simulink model "c00008_harness"  (R2018a)
settings: Solver=FixedStepAuto  StartTime=0  StopTime=300  FixedStep=0.01  RelTol=1e-3
undefined symbols (not defined in the file): sigbuilder_block
settings Model: SldvGeneratedHarnessModel=TestUnitModel=Tanks150|  Creator=aarrieta  LastModifiedBy=umarkiegi
settings DataIOCC: ExternalInput=externalinputdata  SaveFormat=StructureWithTime
settings DebuggingCC: InheritedTsInSrcMsg=none
settings ConfigComp: CovEnable=on  CovScope=ReferencedModels  RecordCoverage=on  CovMetricSettings=dcmobe  CovHTMLOptions=-aTS=1 -bRG=1 -bTC=0 -hTR=0 -nFC=0 -scm=1 -bcm=1  CovHtmlReporting=on

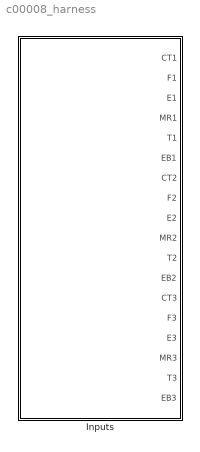
== system c00008_harness ==
  Inputs : Subsystem  Tag=STV Subsys  LoadFcn=sigbuilder_block('load');  StartFcn=sigbuilder_block('start');  StopFcn=sigbuilder_block('stop');  ClipboardFcn=sigbuilder_block('clipboard');  mask(Sigbuilder block){tuvar=[0:10]}
      mask init:
      | if ~strcmp(get_param(bdroot(gcb),'SimulationStatus'),'stopped'),tuvar = sigbuilder_block('maskInit'); end
      settings: CopyFcn=sigbuilder_block('copy');  DeleteFcn=sigbuilder_block('delete');  ModelCloseFcn=sigbuilder_block('modelClose');  PreSaveFcn=sigbuilder_block('preSave');  PauseFcn=sigbuilder_block('pause');  ContinueFcn=sigbuilder_block('continue');  NameChangeFcn=sigbuilder_block('namechange');  OpenFcn=sigbuilder_block('open',[276.75 163.5 675.75 486.75 ]);  CloseFcn=sigbuilder_block('close');
      mask Display: plot(0, 0, 100, 100,[2, 2, 32, 32, 2], [68, 8, 8, 68, 68],[32, 2], [38, 38], [32, 19, 2],[53, 60, 44], [32, 17, 17, 2],[16, 16, 31, 31]);txt = getActiveGroup(gcbh);text(2, 100, txt,'verticalAlignment', 'top');

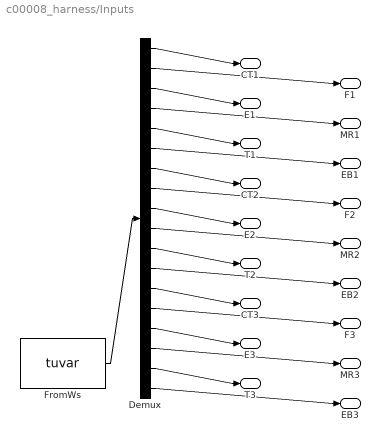
== system c00008_harness/Inputs ==
  Demux : Demux  Tag=STV Demux  Outputs=18
  FromWs : FromWorkspace  Tag=STV FromWs  VariableName=tuvar  SampleTime=0
  CT1 : Outport  Tag=STV Outport
  F1 : Outport  Tag=STV Outport  Port=2
  E1 : Outport  Tag=STV Outport  Port=3
  MR1 : Outport  Tag=STV Outport  Port=4
  T1 : Outport  Tag=STV Outport  Port=5
  EB1 : Outport  Tag=STV Outport  Port=6
  CT2 : Outport  Tag=STV Outport  Port=7
  F2 : Outport  Tag=STV Outport  Port=8
  E2 : Outport  Tag=STV Outport  Port=9
  MR2 : Outport  Tag=STV Outport  Port=10
  T2 : Outport  Tag=STV Outport  Port=11
  EB2 : Outport  Tag=STV Outport  Port=12
  CT3 : Outport  Tag=STV Outport  Port=13
  F3 : Outport  Tag=STV Outport  Port=14
  E3 : Outport  Tag=STV Outport  Port=15
  MR3 : Outport  Tag=STV Outport  Port=16
  T3 : Outport  Tag=STV Outport  Port=17
  EB3 : Outport  Tag=STV Outport  Port=18
  wires:
  FromWs/1 -> Demux/1
  Demux/1 -> CT1/1
  Demux/2 -> F1/1
  Demux/3 -> E1/1
  Demux/4 -> MR1/1
  Demux/5 -> T1/1
  Demux/6 -> EB1/1
  Demux/7 -> CT2/1
  Demux/8 -> F2/1
  Demux/9 -> E2/1
  Demux/10 -> MR2/1
  Demux/11 -> T2/1
  Demux/12 -> EB2/1
  Demux/13 -> CT3/1
  Demux/14 -> F3/1
  Demux/15 -> E3/1
  Demux/16 -> MR3/1
  Demux/17 -> T3/1
  Demux/18 -> EB3/1
